simulink model "11_3"  (R2018b)
settings: Solver=VariableStepAuto  StartTime=0.0  StopTime=2  MaxStep=0.01  RelTol=1e-3
values from neighbouring files (symbols this model uses):
  A = [0 1; 4 0]    [K_and_M_finder.m]    (also in Lf_and_Mf_finder.m; Output_Mf_Lf.m; solver.m)
  B = [1; 1]    [K_and_M_finder.m]    (also in Lf_and_Mf_finder.m; Output_Mf_Lf.m; solver.m)
  C = [3 0]    [Lf_and_Mf_finder.m]    (also in Output_Mf_Lf.m; solver.m)
  D = 3    [Lf_and_Mf_finder.m]    (also in Output_Mf_Lf.m; solver.m)
  G_sh = [0 -(16/3)^2; 1 -32/3]    [Output_Mf_sh.m]    (also in solver.m)
  Gf = [0 1; -9 0]    [Lf_and_Mf_finder.m]    (also in Mn_and_L_finder.m; Output_Mf_Lf.m; Output_Mf_sh.m)
  Hf = [1 0]    [Lf_and_Mf_finder.m]    (also in Mn_and_L_finder.m; Output_Mf_Lf.m; Output_Mf_sh.m)
  Kk = [k1Sol k2Sol]    [K_and_M_finder.m]
  L_sh = transpose(-Hn_sh * inv(Mn))    [Mn_and_L_finder.m]    (also in Output_Mf_sh.m = [0; 1]; solver.m = [0; 1])
  Lf_O = [l1Sol l2Sol]    [Output_Mf_Lf.m]
  Mf_sh = sylv(-G_sh,Gf,L_sh.*Hf)    [Output_Mf_sh.m]
settings Model: Creator=kekos  LastModifiedBy=kekos

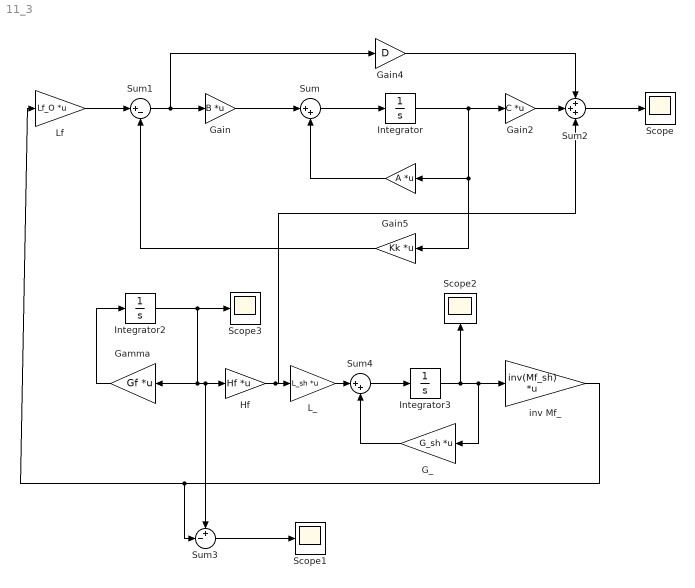
== system 11_3 ==
  " " : Gain  Gain=A  Multiplication=Matrix(K*u)
  " G_" : Gain  Gain=G_sh  Multiplication=Matrix(K*u)
  Gain : Gain  Gain=B  Multiplication=Matrix(K*u)
  Gain2 : Gain  Gain=C  Multiplication=Matrix(K*u)
  Gain4 : Gain  Gain=D
  Gain5 : Gain  Gain=Kk  Multiplication=Matrix(K*u)
  Gamma : Gain  Gain=Gf  Multiplication=Matrix(K*u)
  Hf : Gain  Gain=Hf  Multiplication=Matrix(K*u)
  Integrator : Integrator
  Integrator2 : Integrator  InitialCondition=[-2.91; -19.1]
  Integrator3 : Integrator
  L_ : Gain  Gain=L_sh  Multiplication=Matrix(K*u)
  "Lf " : Gain  Gain=Lf_O  Multiplication=Matrix(K*u)
  Scope{,1..3} (4 alike) : Scope
  Sum : Sum  Inputs=|++
  Sum1 : Sum  Inputs=|+-
  Sum2 : Sum  Inputs=+++
  Sum3 : Sum  Inputs=+-|
  Sum4 : Sum  Inputs=|++
  inv Mf_ : Gain  Gain=inv(Mf_sh)  Multiplication=Matrix(K*u)
  wires:
  Gain4/1 -> Sum2/1
  Gamma/1 -> Integrator2/1
  " "/1 -> Sum/2
  "Lf "/1 -> Sum1/1
  Gain2/1 -> Sum2/2
  Integrator/1 -> Gain2/1, " "/1, Gain5/1
  Sum2/1 -> Scope/1
  Gain5/1 -> Sum1/2
  Sum/1 -> Integrator/1
  Gain/1 -> Sum/1
  Sum1/1 -> Gain4/1, Gain/1
  Integrator2/1 -> Scope3/1, Hf/1, Sum3/1, Gamma/1
  Integrator3/1 -> " G_"/1, inv Mf_/1, Scope2/1
  L_/1 -> Sum4/1
  " G_"/1 -> Sum4/2
  Sum4/1 -> Integrator3/1
  inv Mf_/1 -> Sum3/2, "Lf "/1
  Hf/1 -> Sum2/3, L_/1
  Sum3/1 -> Scope1/1
